simulink model "ostim_prosesNonlinearClosedLoop"  (R2021b)
settings: Solver=FixedStepAuto  StartTime=0.0  StopTime=20000  FixedStep=1  RelTol=1e-3
settings Model: Creator=ismt  LastModifiedBy=ismt

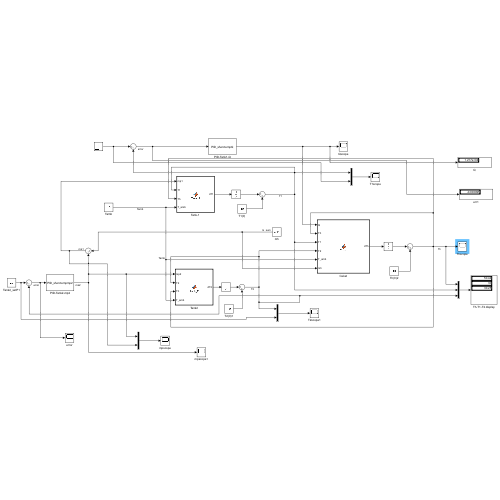
[thumbnail: Simulink's stored preview of the top-level diagram]
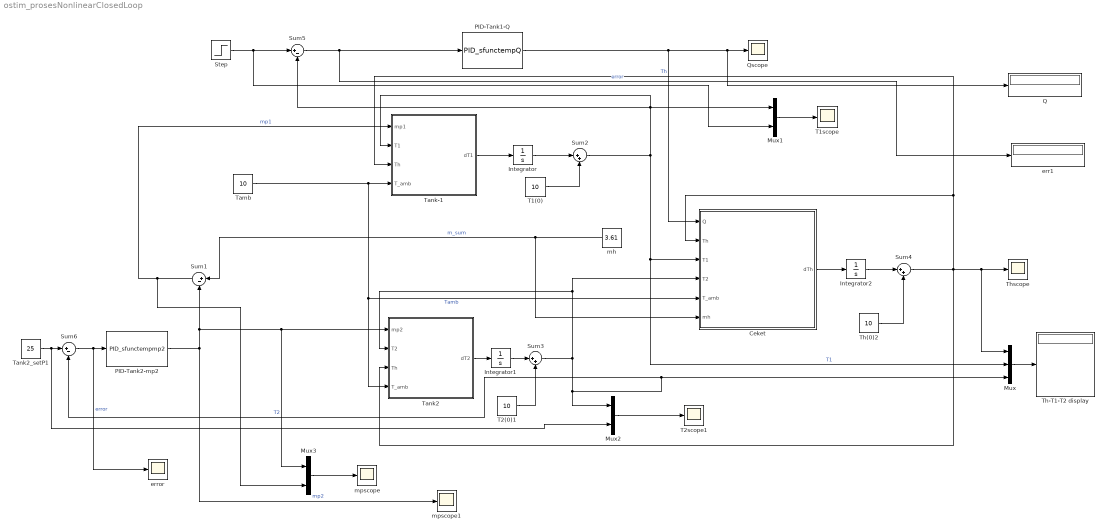
== system ostim_prosesNonlinearClosedLoop ==
  Ceket : MATLAB Function  TreatAsAtomicUnit=on
  Integrator : Integrator
  Integrator1 : Integrator
  Integrator2 : Integrator
  Mux : Mux  Inputs=3
  Mux1 : Mux  Inputs=2
  Mux2 : Mux  Inputs=2
  Mux3 : Mux  Inputs=2
  PID-Tank1-Q : S-Function  FunctionName=PID_sfunctempQ  Parameters=KC,TI,TD  SFunctionDeploymentMode=off  EnableBusSupport=off  mask{KC=40000, TI=4000, TD=100}
  PID-Tank2-mp2 : S-Function  FunctionName=PID_sfunctempmp2  Parameters=KC,TI,TD  SFunctionDeploymentMode=off  EnableBusSupport=off  mask{KC=15, TI=1000, TD=2}
  Q : Display
  Qscope : Scope
  Step : Step  Time=10000  Before=25  After=30  SampleTime=0
  Sum1 : Sum  Inputs=|+-
  Sum2 : Sum  Inputs=|++
  Sum3 : Sum  Inputs=|++
  Sum4 : Sum  Inputs=|++
  Sum5 : Sum  Inputs=|+-
  Sum6 : Sum  Inputs=|+-
  T1(0) : Constant  Value=10
  T1scope : Scope
  T2(0)1 : Constant  Value=10
  T2scope1 : Scope
  Tamb : Constant  Value=10
  "Tank-1 " : MATLAB Function  TreatAsAtomicUnit=on
  Tank2 : MATLAB Function  TreatAsAtomicUnit=on
  Tank2_setP1 : Constant  Value=25
  Th(0)2 : Constant  Value=10
  Th-T1-T2 display : Display
  Thscope : Scope
  err1 : Display
  error : Scope
  mh : Constant  Value=3.61
  mpscope : Scope
  mpscope1 : Scope
  wires:
  "Tank-1 "/1(dT1) -> Integrator/1
  Integrator/1 -> Sum2/1
  T1(0)/1 -> Sum2/2
  Sum2/1 -> Mux1/1, Sum5/2, "Tank-1 "/2(T1), Mux/2, Ceket/3(T1)  "T1"
  mh/1 -> Ceket/6(mh), Sum1/1  "m_sum"
  Tamb/1 -> Tank2/4(T_amb), Ceket/5(T_amb), "Tank-1 "/4(T_amb)  "Tamb"
  Tank2/1(dT2) -> Integrator1/1
  T2(0)1/1 -> Sum3/2
  Integrator1/1 -> Sum3/1
  Ceket/1(dTh) -> Integrator2/1
  Integrator2/1 -> Sum4/1
  Th(0)2/1 -> Sum4/2
  Sum4/1 -> Tank2/3(Th), "Tank-1 "/3(Th), Ceket/2(Th), Mux/1, Thscope/1  "Th"
  Sum3/1 -> Mux2/1, Mux/3, Sum6/2, Tank2/2(T2), Ceket/4(T2)  "T2"
  Mux/1 -> Th-T1-T2 display/1
  Step/1 -> Mux1/2, Sum5/1
  Sum5/1 -> err1/1, PID-Tank1-Q/1  "error"
  PID-Tank1-Q/1 -> Q/1, Qscope/1, Ceket/1(Q)
  PID-Tank2-mp2/1 -> mpscope1/1, Sum1/2, Mux3/1, Tank2/1(mp2)  "mp2"
  Sum1/1 -> Mux3/2, "Tank-1 "/1(mp1)  "mp1"
  Tank2_setP1/1 -> Mux2/2, Sum6/1
  Sum6/1 -> error/1, PID-Tank2-mp2/1  "error"
  Mux1/1 -> T1scope/1
  Mux2/1 -> T2scope1/1
  Mux3/1 -> mpscope/1

== matlab function ostim_prosesNonlinearClosedLoop/Tank2 ==
  data: mp2 input; T2 input; dT2 output; Th input; T_amb input
function dT2 = Tank_2(mp2,T2,Th,T_amb)
r_tank2 = 0.47; %m
h_tank2 = 0.7; %m
AT2_surf = 2*pi*r_tank2*h_tank2; %m^2
ht2 = 100; %(J/s*m^2*K)
m_tank2 = 468; %kg;
cp_fluid = 4.18*1000; %(J/kg*K);
cp_tank = cp_fluid; %tank1,2 ile soğutma sıvısı aynı kabulü ile
Tc2 = T2 - ((T2-Th)*exp((-ht2*AT2_surf)/(mp2*cp_fluid)));
dT2 = (mp2*cp_fluid)/(cp_tank*m_tank2)*(Th-Tc2) - (ht2*AT2_surf*(T2-T_amb))/(m_tank2*cp_tank);

== matlab function ostim_prosesNonlinearClosedLoop/Tank-1  ==
  data: mp1 input; T1 input; dT1 output; Th input; T_amb input
function dT1 = Tank_1(mp1,T1,Th,T_amb)

r_tank1 = 0.55; %m
h_tank1 = 0.99+(0.17/2); %m
AT1_surf = 2*pi*r_tank1*h_tank1; %m^2
ht1 = 100; %(J/s*m^2*K)
cp_fluid = 4.18*1000; %(J/kg*K);
cp_tank = cp_fluid; %tank1,2 ile soğutma sıvısı aynı kabulü ile
m_tank1 = 1000; %kg;
Tc1 = T1 - ((T1-Th)*exp((-ht1*AT1_surf)/(mp1*cp_fluid)));
dT1 = (mp1*cp_fluid)/(cp_tank*m_tank1)*(Th-Tc1) - (ht1*AT1_surf*(T1-T_amb))/(m_tank1*cp_tank);

== matlab function ostim_prosesNonlinearClosedLoop/Ceket ==
  data: Q input; Th input; T1 input; T2 input; dTh output; T_amb input; mh input
function dTh = Ceket(Q,Th,T1,T2,T_amb,mh)

uRes = 10; %(J/s*m^2*K)
A_res = 1; %m^2 bu değer seçildi.. Sorulabilir
cp_fluid = 4.18*1000; %(J/kg*K);
ht1 = 100; %(J/s*m^2*K)
r_tank1 = 0.55; %m
h_tank1 = 0.99+(0.17/2); %m
AT1_surf = 2*pi*r_tank1*h_tank1; %m^2
r_tank2 = 0.47; %m
h_tank2 = 0.7; %m

AT2_surf = 2*pi*r_tank2*h_tank2; %m^2
ht2 = 100; %(J/s*m^2*K)
V1 = Q/(mh*cp_fluid);
V2 = -(uRes*A_res)/(mh*cp_fluid);
V3 = -(ht1*AT1_surf)/(mh*cp_fluid);
V4 = -(ht2*AT2_surf)/(mh*cp_fluid);
dTh = V1 + V2*(Th-T_amb) + V3*(Th-T1) + V4*(Th-T2);
